simulink model "Ford_T3T6_ArchCnctnDigrm"  (R2016b)
settings: Solver=FixedStepDiscrete  StartTime=0.0  StopTime=10.0  RelTol=1e-3  EnableMultiTasking=on
libraries: canmsglib x15
(part 15 of 15)

== system Ford_T3T6_ArchCnctnDigrm/Monitor System/Measured Signals/ProcessHandwheelTorqueSignal/ES229C_HwTqCorrln ==
  HwTqA : Inport
  HwTqAQlfr : Inport  Port=2
  HwTqARollgCntr : Inport  Port=3
  HwTqB : Inport  Port=4
  HwTqBQlfr : Inport  Port=5
  HwTqBRollgCntr : Inport  Port=6
  HwTqC : Inport  Port=7
  HwTqCQlfr : Inport  Port=8
  HwTqCRollgCntr : Inport  Port=9
  HwTqD : Inport  Port=10
  HwTqDQlfr : Inport  Port=11
  HwTqDRollgCntr : Inport  Port=12
  FltInj_u08 : Inport  Port=13
  GetNtcQlfrSts : Inport  Port=14
  SetNtcSts : Inport  Port=15
  HwTqCorrlnSts : Outport
  HwTqIdptSig : Outport  Port=2

== system Ford_T3T6_ArchCnctnDigrm/Vehicle Com/Rx Messages/Acc Pedal Posn/MM062A_FordMsg204BusHiSpd ==
  AccrPedlPosnSts : Inport
  AccrPedlPosnStsQlyFac : Inport  Port=2
  CanDtcInhb : Inport  Port=3
  EngSpd : Inport  Port=4
  EpsLifeCycMod : Inport  Port=5
  TrlrBackUpAssiEnad : Inport  Port=6
  GetRefTmr100MicroSec32bit : Inport  Port=7
  GetTiSpan100MicroSec32bit : Inport  Port=8
  SetNtcSts : Inport  Port=9
  FordVehAccrPedlPosnStsQlyFac : Outport
  FordVehAccrPedlPosnStsQlyFacRaw : Outport  Port=2
  FordVehAccrPedlPosnStsRaw : Outport  Port=3
  FordVehAccrPedlPosnStsVld : Outport  Port=4
  FordVehEngSpdRaw : Outport  Port=5
  FordVehEngSpdVld : Outport  Port=6
  FordMsg204HiSpdBusClrDiagcSrv : Outport  Port=7
  FordMsg204HiSpdBusSerlComInpDi : Outport  Port=8

== system Ford_T3T6_ArchCnctnDigrm/Vehicle Com/Rx Messages/Ambient Temperature/MM078A_FordMsg41ABusHiSpd ==
  ClrDiagcFlgProxy : Inport
  FordCanDtcInhb : Inport  Port=2
  FordEpsLifeCycMod : Inport  Port=3
  Ford_Outside_Air_Temp_Stat : Inport  Port=4
  GetRefTmr100MicroSec32bit : Inport  Port=5
  GetTiSpan100MicroSec32bit : Inport  Port=6
  SetNtcSts : Inport  Port=7
  FordVehOutdAirT : Outport
  FordVehOutdAirTRaw : Outport  Port=2
  ComIPduCallout_Climate_Control_Data_FD1 : Outport  Port=3
  ComTimeoutNotification_Outside_Air_Temp_Stat : Outport  Port=4

== system Ford_T3T6_ArchCnctnDigrm/Vehicle Com/Rx Messages/Brake Data/MM052A_FordMsg07DBusHiSpd ==
  ClrDiagcFlgProxy : Inport
  FordBrkOscnRednEnad : Inport  Port=2
  FordCanDtcInhb : Inport  Port=3
  FordEpsLifeCycMod : Inport  Port=4
  FordTrlrBackUpAssiEnad : Inport  Port=5
  Ford_BrkTot_Tq_Actl : Inport  Port=6
  Ford_VehVertComp_A_Actl : Inport  Port=7
  GetRefTmr100MicroSec32bit : Inport  Port=8
  GetTiSpan100MicroSec32bit : Inport  Port=9
  SetNtcSts : Inport  Port=10
  FordVehActBrkTqRaw : Outport
  FordVehBrkTqVld : Outport  Port=2
  FordVehVertACmpdRaw : Outport  Port=3
  FordVehVertAVld : Outport  Port=4
  ComIPduCallout_BrakeSnData_4_FD1 : Outport  Port=5
  ComTimeoutNotification_BrkTot_Tq_Actl : Outport  Port=6

== system Ford_T3T6_ArchCnctnDigrm/Vehicle Com/Rx Messages/Brake Data/MM058A_FordMsg165BusHiSpd ==
  ClrDiagcFlgProxy : Inport
  FordCanDtcInhb : Inport  Port=2
  FordEpsLifeCycMod : Inport  Port=3
  FordTrlrBackupAssiEnad : Inport  Port=4
  Ford_BpedDrvAppl_D_Actl1 : Inport  Port=5
  Ford_BpedDrvAppl_D_Qf1 : Inport  Port=6
  GetRefTmr100MicroSec32bit : Inport  Port=7
  GetTiSpan100MicroSec32bit : Inport  Port=8
  SetNtcSts : Inport  Port=9
  FordVehBrkPedlAppld : Outport
  FordVehBrkPedlAppldQlyFac : Outport  Port=2
  FordVehBrkPedlVld : Outport  Port=3
  ComIPduCallout_EngBrakeData_FD1 : Outport  Port=4
  ComTimeoutNotification_BpedDrvAppl_D_Actl : Outport  Port=5

== system Ford_T3T6_ArchCnctnDigrm/Vehicle Com/Rx Messages/Brake Data/MM063A_FordMsg213BusHiSpd ==
  ClrDiagcFlgProxy : Inport
  FordBrkOscnRednEnad : Inport  Port=2
  FordCanDtcInhb : Inport  Port=3
  FordEpsLifeCycMod : Inport  Port=4
  FordEvasSteerAssiEnad : Inport  Port=5
  FordLaneCentrAssiEnad : Inport  Port=6
  FordLaneDetnWarnEnad : Inport  Port=7
  FordLkaEnad : Inport  Port=8
  FordTrfcJamAssiEnad : Inport  Port=9
  Ford_AbsActv_B_Actl1 : Inport  Port=10
  Ford_CmbbBrkDis_B_Actl1 : Inport  Port=11
  Ford_CmbbDeny_B_ActlBrk1 : Inport  Port=12
  Ford_StabCtlBrkActv_B_Actl1 : Inport  Port=13
  GetRefTmr100MicroSec32bit : Inport  Port=14
  GetTiSpan100MicroSec32bit : Inport  Port=15
  SetNtcSts : Inport  Port=16
  FordVehAbsActv : Outport
  FordVehAbsEscStsVld : Outport  Port=2
  FordVehCllsnMtgtnByBrkgDenied : Outport  Port=3
  FordVehCllsnMtgtnByBrkgDisad : Outport  Port=4
  FordVehEscActv : Outport  Port=5
  ComIPduCallout_DesiredTorqBrk_FD1 : Outport  Port=6
  ComTimeoutNotification_CmbbDeny_B_ActlBrk : Outport  Port=7

== system Ford_T3T6_ArchCnctnDigrm/Vehicle Com/Rx Messages/Brake Data/MM077A_FordMsg415BusHiSpd ==
  ClrDiagcFlgProxy : Inport
  FordAbsPrsnt : Inport  Port=2
  FordCanDtcInhb : Inport  Port=3
  FordEpsLifeCycMod : Inport  Port=4
  FordTrlrBackupAssiEnad : Inport  Port=5
  Ford_LsmcBrkDecel_D_Stat1 : Inport  Port=6
  Ford_VehVActlBrk_D_Qf1 : Inport  Port=7
  Ford_VehVActlBrk_No_Cnt : Inport  Port=8
  Ford_VehVActlBrk_No_Cs : Inport  Port=9
  Ford_Veh_V_ActlBrk : Inport  Port=10
  GetRefTmr100MicroSec32bit : Inport  Port=11
  GetTiSpan100MicroSec32bit : Inport  Port=12
  SetNtcSts : Inport  Port=13
  FordVehLoSpdMtnCtrlBrkSprtSts : Outport
  FordVehLoSpdMtnCtrlBrkSprtStsRaw : Outport  Port=2
  FordVehLoSpdMtnCtrlBrkSprtVld : Outport  Port=3
  FordVehSpdBrkModl : Outport  Port=4
  FordVehSpdBrkModlLoQlyVld : Outport  Port=5
  FordVehSpdBrkModlRaw : Outport  Port=6
  FordVehSpdBrkModlVld : Outport  Port=7
  FordVehSpdChksBrkModl : Outport  Port=8
  FordVehSpdCntrBrkModl : Outport  Port=9
  FordVehSpdQlyFacBrkModl : Outport  Port=10
  ComIPduCallout_BrakeSysFeatures_FD1 : Outport  Port=11
  ComTimeoutNotification_Veh_V_ActlBrk : Outport  Port=12

== system Ford_T3T6_ArchCnctnDigrm/Vehicle Com/Rx Messages/Evasive Steer Assist/MM075A_FordMsg3D7BusHiSpd ==
  ClrDiagcFlgProxy : Inport
  FordCanDtcInhb : Inport  Port=2
  FordEpsLifeCycMod : Inport  Port=3
  FordEvasSteerAssiEnad : Inport  Port=4
  Ford_CmbbObjClass_D_Stat1 : Inport  Port=5
  Ford_CmbbObjColl_T_Actl : Inport  Port=6
  Ford_CmbbObjConfdnc_D_Stat1 : Inport  Port=7
  Ford_CmbbObjDistLat_L_Actl : Inport  Port=8
  Ford_CmbbObjDistLong_L_Actl : Inport  Port=9
  Ford_CmbbObjRelLat_V_Actl : Inport  Port=10
  Ford_CmbbObjRelLong_V_Actl : Inport  Port=11
  Ford_EsaEnbl_D2_Rq1 : Inport  Port=12
  GetRefTmr100MicroSec32bit : Inport  Port=13
  GetTiSpan100MicroSec32bit : Inport  Port=14
  SetNtcSts : Inport  Port=15
  FordVehCllsnMtgtnByBrkgLatDstRaw : Outport
  FordVehCllsnMtgtnByBrkgLgtDstRaw : Outport  Port=2
  FordVehCllsnMtgtnByBrkgObjDataConfLvlRaw : Outport  Port=3
  FordVehCllsnMtgtnByBrkgObjTypClassnRaw : Outport  Port=4
  FordVehCllsnMtgtnByBrkgRelLatVelRaw : Outport  Port=5
  FordVehCllsnMtgtnByBrkgRelLgtVelRaw : Outport  Port=6
  FordVehCllsnMtgtnByBrkgTiToCllsnRaw : Outport  Port=7
  FordVehEvasSteerAssiEnadReqRaw : Outport  Port=8
  FordVehEvasSteerAssiImgProcrModlAVld : Outport  Port=9
  ComIPduCallout_Steer_Assist_Data_FD1 : Outport  Port=10
  ComTimeoutNotification_EsaEnbl_D2_Rq : Outport  Port=11

== system Ford_T3T6_ArchCnctnDigrm/Vehicle Com/Rx Messages/Evasive Steer Assist/MM134A_FordMsg2FDBusHiSpd ==
  ClrDiagcFlgProxy : Inport
  FordCanDtcInhb : Inport  Port=2
  FordEpsLifeCycMod : Inport  Port=3
  FordInvldMsgDiagcInhb : Inport  Port=4
  FordMfgDiagcInhb : Inport  Port=5
  FordMissMsgDiagcInhb : Inport  Port=6
  FordTrlrBackupAssiEnad : Inport  Port=7
  Ford_EsaOn_B_Rq : Inport  Port=8
  GetRefTmr100MicroSec32bit : Inport  Port=9
  GetTiSpan100MicroSec32bit : Inport  Port=10
  SetNtcSts : Inport  Port=11
  FordVehEvasSteerAssiReq : Outport
  FordVehEvasSteerAssiReqVld : Outport  Port=2
  ComIPduCallout_Mc_Send_Signals_2_FD1 : Outport  Port=3
  ComTimeoutNotification_EsaOn_B_Rq : Outport  Port=4

== system Ford_T3T6_ArchCnctnDigrm/Vehicle Com/Rx Messages/Lane Keep Asssist/MM073A_FordMsg3CABusHiSpd ==
  ClrDiagcFlgProxy : Inport
  FordCanDtcInhb : Inport  Port=2
  FordEpsLifeCycMod : Inport  Port=3
  FordLaneDetnWarnEnad : Inport  Port=4
  FordLaneKeepAssiEnad : Inport  Port=5
  Ford_LaCurvature_No_Calc : Inport  Port=6
  Ford_LaRampType_B_Req1 : Inport  Port=7
  Ford_LaRefAng_No_Req : Inport  Port=8
  Ford_LdwActvIntns_D_Req1 : Inport  Port=9
  Ford_LdwActvStats_D_Req1 : Inport  Port=10
  Ford_LkaActvStats_D2_Req1 : Inport  Port=11
  GetRefTmr100MicroSec32bit : Inport  Port=12
  GetTiSpan100MicroSec32bit : Inport  Port=13
  SetNtcSts : Inport  Port=14
  FordVehLaneAssiImgProcgModlAVld : Outport
  FordVehLaneDetnWarnInten : Outport  Port=2
  FordVehLaneDetnWarnSts : Outport  Port=3
  FordVehLaneKeepSysCrvt : Outport  Port=4
  FordVehLaneKeepSysCrvtRaw : Outport  Port=5
  FordVehLaneKeepSysRampTyp : Outport  Port=6
  FordVehLaneKeepSysReqdAg : Outport  Port=7
  FordVehLaneKeepSysReqdAgRaw : Outport  Port=8
  FordVehLaneKeepSysSts : Outport  Port=9
  ComIPduCallout_Lane_Assist_Data1_FD1 : Outport  Port=10
  ComTimeoutNotification_LaCurvature_No_Calc : Outport  Port=11

== system Ford_T3T6_ArchCnctnDigrm/Vehicle Com/Rx Messages/Lat and Long Acceleration/MM074A_FordMsg3D3BusHiSpd ==
  CanDtcInhb : Inport
  EpsLifeCycMod : Inport  Port=2
  LaneCentrAssiEnad : Inport  Port=3
  LatCtrlCrvt : Inport  Port=4
  LatCtrlCrvtRate : Inport  Port=5
  LatCtrlHandsOffDetnTqStimlsReq : Inport  Port=6
  LatCtrlPah : Inport  Port=7
  LatCtrlPahOffs : Inport  Port=8
  LatCtrlPrcsn : Inport  Port=9
  LatCtrlRampTyp : Inport  Port=10
  LatCtrlReq : Inport  Port=11
  LatCtrlRingMax : Inport  Port=12
  MissMsg3D3TiFlg : Inport  Port=13
  TrfcJamAssiEnad : Inport  Port=14
  GetRefTmr100MicroSec32bit : Inport  Port=15
  GetTiSpan100MicroSec32bit : Inport  Port=16
  SetNtcSts : Inport  Port=17
  FordVehLatCtrlCrvt : Outport
  FordVehLatCtrlCrvtRate : Outport  Port=2
  FordVehLatCtrlCrvtRateRaw : Outport  Port=3
  FordVehLatCtrlCrvtRaw : Outport  Port=4
  FordVehLatCtrlHandsOffDetnTqStimlsReq : Outport  Port=5
  FordVehLatCtrlImgProcrModlAVld : Outport  Port=6
  FordVehLatCtrlPah : Outport  Port=7
  FordVehLatCtrlPahOffs : Outport  Port=8
  FordVehLatCtrlPahOffsRaw : Outport  Port=9
  FordVehLatCtrlPahRaw : Outport  Port=10
  FordVehLatCtrlPrcsn : Outport  Port=11
  FordVehLatCtrlRampTyp : Outport  Port=12
  FordVehLatCtrlReq : Outport  Port=13
  FordVehLatCtrlRingMax : Outport  Port=14
  FordMsg3D3HiSpdBusClrDiagcSrv : Outport  Port=15
  FordMsg3D3HiSpdBusSerlComInpDi : Outport  Port=16

== system Ford_T3T6_ArchCnctnDigrm/Vehicle Com/Rx Messages/Lat and Long Acceleration/MM124A_FordMsg077BusHiSpd1 ==
  FordBrkOscnRednEnad : Inport
  FordCanDtcInhb : Inport  Port=2
  FordEpsLifeCycMod : Inport  Port=3
  FordEvasSteerAssiEnad : Inport  Port=4
  FordLaneKeepingAssiEnad : Inport  Port=5
  FordMissMsgDiagcInhb : Inport  Port=6
  FordPullDriftCmpEnad : Inport  Port=7
  FordTqSteerCmpEnad : Inport  Port=8
  FordTrlrBackupAssiEnad : Inport  Port=9
  Ford_VehLatComp_A_Actl : Inport  Port=10
  Ford_VehLongComp_A_Actl : Inport  Port=11
  Ford_VehOverGnd_V_Est : Inport  Port=12
  Ford_VehYawComp_W_Actl : Inport  Port=13
  LaneCentrAssiEnad : Inport  Port=14
  TrfcJamAssiEnad : Inport  Port=15
  GetRefTmr100MicroSec32bit : Inport  Port=16
  GetTiSpan100MicroSec32bit : Inport  Port=17
  SetNtcSts : Inport  Port=18
  FordVehLatACmpd : Outport
  FordVehLatACmpdRaw : Outport  Port=2
  FordVehLatACmpdVld : Outport  Port=3
  FordVehLgtACmpd : Outport  Port=4
  FordVehLgtACmpdRaw : Outport  Port=5
  FordVehLgtACmpdVld : Outport  Port=6
  FordVehSpdOverGnd : Outport  Port=7
  FordVehSpdOverGndRaw : Outport  Port=8
  FordVehSpdOverGndVld : Outport  Port=9
  FordVehYawRateCmpd : Outport  Port=10
  FordVehYawRateCmpdRaw : Outport  Port=11
  FordVehYawRateCmpdVld : Outport  Port=12
  ComIPduCallout_BrakeSnData_3_FD1 : Outport  Port=13
  ComTimeoutNotification_VehLatComp_A_Actl : Outport  Port=14

== system Ford_T3T6_ArchCnctnDigrm/Vehicle Com/Rx Messages/Park Assist/MM071A_FordMsg3A8BusHiSpd ==
  ClrDiagcFlgProxy : Inport
  FordApaEnad : Inport  Port=2
  FordCanDtcInhb : Inport  Port=3
  FordEpsLifeCycMod : Inport  Port=4
  FordExtAgCtrlEnad : Inport  Port=5
  FordTrlrBackUpAssiEnad : Inport  Port=6
  Ford_ApaSys_D_Stat1 : Inport  Port=7
  Ford_EPASExtAngleStatReq1 : Inport  Port=8
  Ford_ExtSteeringAngleReq2 : Inport  Port=9
  GetRefTmr100MicroSec32bit : Inport  Port=10
  GetTiSpan100MicroSec32bit : Inport  Port=11
  SetNtcSts : Inport  Port=12
  FordVehParkAidModlReqdAg : Outport
  FordVehParkAidModlReqdAgRaw : Outport  Port=2
  FordVehParkAidModlReqdAgVldInt : Outport  Port=3
  FordVehParkAidModlReqdSts : Outport  Port=4
  FordVehParkAidModlStsVld : Outport  Port=5
  FordVehParkAidModlStsVldInt : Outport  Port=6
  FordVehParkAidModlSysSt : Outport  Port=7
  ComIPduCallout_ParkAid_Data_FD1 : Outport  Port=8
  ComTimeoutNotification_EPASExtAngleStatReq : Outport  Port=9

== system Ford_T3T6_ArchCnctnDigrm/Vehicle Com/Rx Messages/Pinion Data/MM070A_FordMsg414BusHiSpd ==
  Ford_StePinOffst_An_Est : Inport
  Ford_StePinOffst_D_Stat1 : Inport  Port=2
  Ford_StePinOffst_No_Cnt : Inport  Port=3
  Ford_StePinOffst_No_Cs : Inport  Port=4
  GetRefTmr100MicroSec32bit : Inport  Port=5
  GetTiSpan100MicroSec32bit : Inport  Port=6
  FordVehSteerPinionAgOffs : Outport
  FordVehSteerPinionAgOffsRaw : Outport  Port=2
  FordVehSteerPinionAgOffsVld : Outport  Port=3
  FordVehSteerPinionOffsChks : Outport  Port=4
  FordVehSteerPinionOffsCnt : Outport  Port=5
  FordVehSteerPinionOffsSts : Outport  Port=6
  FordVehSteerPinionOffsStsRaw : Outport  Port=7
  ComIPduCallout_BrakeSnData_6_HS2 : Outport  Port=8
  ComTimeoutNotification_Ford_StePinOffst_D_Stat : Outport  Port=9

== system Ford_T3T6_ArchCnctnDigrm/Vehicle Com/Rx Messages/Steering Request Command/MM123A_FordMsg076BusHiSpd1 ==
  ClrDiagcFlgProxy : Inport
  DrvrSteerRcmdnEnad : Inport  Port=2
  FordCanDtcInhb : Inport  Port=3
  FordEpsLifeCycMod : Inport  Port=4
  Ford_DrvSte_D_Stat : Inport  Port=5
  Ford_DrvSte_Tq_Rq : Inport  Port=6
  GetRefTmr100MicroSec32bit : Inport  Port=7
  GetTiSpan100MicroSec32bit : Inport  Port=8
  SetNtcSts : Inport  Port=9
  FordVehDrvrSteerReqCmd : Outport
  FordVehDrvrSteerReqCmdVld : Outport  Port=2
  FordVehDrvrSteerReqSts : Outport  Port=3
  ComIPduCallout_BrakeSnData_5_FD1 : Outport  Port=4
  ComTimeoutNotification_DrvSte_Tq_Rq : Outport  Port=5

== system Ford_T3T6_ArchCnctnDigrm/Vehicle Com/Rx Messages/Trailer Aid/MM057A_FordMsg215BusHiSpd ==
  ClrDiagcFlgProxy : Inport
  FordCanDtcInhb : Inport  Port=2
  FordEpsLifeCycMod : Inport  Port=3
  FordTrlrBackupAssiEnad : Inport  Port=4
  Ford_TrlrAidMde_D_Rq1 : Inport  Port=5
  GetRefTmr100MicroSec32bit : Inport  Port=6
  GetTiSpan100MicroSec32bit : Inport  Port=7
  SetNtcSts : Inport  Port=8
  FordVehTrlrAidModReq : Outport
  FordVehTrlrAidModReqVld : Outport  Port=2
  ComIPduCallout_APIM_Send_Signals_2_FD1 : Outport  Port=3
  ComTimeoutNotification_TrlrAidMde_D_Rq : Outport  Port=4

== system Ford_T3T6_ArchCnctnDigrm/Vehicle Com/Rx Messages/Trailer Aid/MM069A_FordMsg3F1BusHiSpd ==
  ClrDiagcFlgProxy : Inport
  FordCanDtcInhb : Inport  Port=2
  FordEpsLifeCycMod : Inport  Port=3
  FordMfgDiagcInhb : Inport  Port=4
  FordMissMsgDiagcInhb : Inport  Port=5
  FordTrlrBackUpAssiEnad : Inport  Port=6
  Ford_TrlrAidCancl_B_Rq1 : Inport  Port=7
  GetRefTmr100MicroSec32bit : Inport  Port=8
  GetTiSpan100MicroSec32bit : Inport  Port=9
  SetNtcSts : Inport  Port=10
  FordVehTrlrAidCnclReq : Outport
  FordVehTrlrAidCnclReqVld : Outport  Port=2
  ComIPduCallout_APIM_Sen_Signals1_FD1 : Outport  Port=3
  ComTimeoutNotification_TrlrAidCancl_B_Rq : Outport  Port=4

== system Ford_T3T6_ArchCnctnDigrm/Vehicle Com/Rx Messages/Trailer Aid/MM080A_FordMsg451BusHiSpd ==
  ClrDiagcFlgProxy : Inport
  FordCanDtcInhb : Inport  Port=2
  FordEpsLifeCycMod : Inport  Port=3
  FordTrlrBackupAssiEnad : Inport  Port=4
  Ford_TrlrRvrseEnbl_D2_Stat1 : Inport  Port=5
  Ford_TrlrRvrseMsgTxt_D2_Rq : Inport  Port=6
  GetRefTmr100MicroSec32bit : Inport  Port=7
  GetTiSpan100MicroSec32bit : Inport  Port=8
  SetNtcSts : Inport  Port=9
  FordVehTrlrRvsEnaRaw : Outport
  FordVehTrlrRvsMsgTxtReqRaw : Outport  Port=2
  ImgProcgDataPrsntInt : Outport  Port=3
  ComIPduCallout_Image_Processing_Data_FD1 : Outport  Port=4
  ComTimeoutNotification_TrlrRvrseMsgTxt_D2_Rq : Outport  Port=5

== system Ford_T3T6_ArchCnctnDigrm/Vehicle Com/Rx Messages/Trailer Aid/MM083A_FordMsg457BusHiSpd ==
  ClrDiagcFlgProxy : Inport
  FordCanDtcInhb : Inport  Port=2
  FordEpsLifeCycMod : Inport  Port=3
  FordTrlrBackupAssiEnad : Inport  Port=4
  Ford_TrlrHitYaw_AnRate_Actl : Inport  Port=5
  Ford_TrlrHitchYaw_An_Actl : Inport  Port=6
  Ford_TrlrHitchYaw_D_Stat1 : Inport  Port=7
  Ford_TrlrYaw_W_Actl : Inport  Port=8
  Ford_TrlrYaw_W_Actl_D_Qf1 : Inport  Port=9
  GetRefTmr100MicroSec32bit : Inport  Port=10
  GetTiSpan100MicroSec32bit : Inport  Port=11
  SetNtcSts : Inport  Port=12
  FordVehTrlrHitchAgRateRaw : Outport
  FordVehTrlrHitchYawAgRaw : Outport  Port=2
  FordVehTrlrHitchYawSts : Outport  Port=3
  FordVehTrlrYawRateQlyFac : Outport  Port=4
  FordVehTrlrYawRateRaw : Outport  Port=5
  ComIPduCallout_TrailerAid_Stat2_FD1 : Outport  Port=6
  ComTimeoutNotification_TrlrHitchYaw_An_Actl : Outport  Port=7

== system Ford_T3T6_ArchCnctnDigrm/Vehicle Com/Rx Messages/Trailer Aid/MM086A_FordMsg443BusHiSpd ==
  ClrDiagcFlgProxy : Inport
  FordCanDtcInhb : Inport  Port=2
  FordEpsLifeCycMod : Inport  Port=3
  FordTrlrBackUpAssiEnad : Inport  Port=4
  Ford_TrlrLampCnnct_B_Actl1 : Inport  Port=5
  GetRefTmr100MicroSec32bit : Inport  Port=6
  GetTiSpan100MicroSec32bit : Inport  Port=7
  SetNtcSts : Inport  Port=8
  FordVehTrlrLampCnctnStsRaw : Outport
  ComIPduCallout_TrailerInfo_FD1 : Outport  Port=2
  ComTimeoutNotification_TrlrLampCnnct_B_Actl : Outport  Port=3

== system Ford_T3T6_ArchCnctnDigrm/Vehicle Com/Rx Messages/Trailer Aid/MM087A_FordMsg445BusHiSpd ==
  ClrDiagcFlgProxy : Inport
  FordCanDtcInhb : Inport  Port=2
  FordEpsLifeCycMod : Inport  Port=3
  FordTrlrBackUpAssiEnad : Inport  Port=4
  Ford_TrlrBrkActCnnct_B_Actl1 : Inport  Port=5
  GetRefTmr100MicroSec32bit : Inport  Port=6
  GetTiSpan100MicroSec32bit : Inport  Port=7
  SetNtcSts : Inport  Port=8
  FordVehTrlrBrkCnctnStsRaw : Outport
  ComIPduCallout_TrailerBrakeInfo_FD1 : Outport  Port=2
  ComTimeoutNotification_TrlrBrkActCnnct_B_Actl : Outport  Port=3

== system Ford_T3T6_ArchCnctnDigrm/Vehicle Com/Rx Messages/Trailer Aid/MM088A_FordMsg45ABusHiSpd ==
  ClrDiagcFlgProxy : Inport
  FordCanDtcInhb : Inport  Port=2
  FordEpsLifeCycMod : Inport  Port=3
  FordTrlrBackupAssiEnad : Inport  Port=4
  Ford_TrlrAnOffstDir_D_Mem1 : Inport  Port=5
  Ford_TrlrAxleToBmpr_L_Actl : Inport  Port=6
  Ford_TrlrIdType_D_Stat1 : Inport  Port=7
  Ford_TrlrId_No_Actl : Inport  Port=8
  Ford_TrlrRvrseCancl_B_Rq1 : Inport  Port=9
  GetRefTmr100MicroSec32bit : Inport  Port=10
  GetTiSpan100MicroSec32bit : Inport  Port=11
  SetNtcSts : Inport  Port=12
  FordVehTrlrAgOffsDirRaw : Outport
  FordVehTrlrAidIdnNrRaw : Outport  Port=2
  FordVehTrlrAxleToBmpRaw : Outport  Port=3
  FordVehTrlrBackupAssiMeasVld : Outport  Port=4
  FordVehTrlrIdnTypRaw : Outport  Port=5
  FordVehTrlrRvsCnclReqRaw : Outport  Port=6
  TrlrAidDataPrsntInt : Outport  Port=7
  ComIPduCallout_TrailerAid_Data_FD1 : Outport  Port=8
  ComTimeoutNotification_TrlrId_No_Actl : Outport  Port=9

== system Ford_T3T6_ArchCnctnDigrm/Vehicle Com/Rx Messages/Trailer Aid/MM090A_FordMsg459BusHiSpd ==
  ClrDiagcFlgProxy : Inport
  FordCanDtcInhb : Inport  Port=2
  FordEpsLifeCycMod : Inport  Port=3
  FordMfgDiagcInhb : Inport  Port=4
  FordMissMsgDiagcInhb : Inport  Port=5
  FordTrlrBackupAssiEnad : Inport  Port=6
  Ford_HitchToVehAxle_L_Calc : Inport  Port=7
  Ford_TrlrAidTrgtId_No_Actl : Inport  Port=8
  Ford_TrlrAid_An3_Actl : Inport  Port=9
  Ford_TrlrAid_AnRate2_Actl : Inport  Port=10
  Ford_TrlrAid_D2_Stat : Inport  Port=11
  Ford_TrlrRvrse_D_Stat : Inport  Port=12
  Ford_TrlrTrgtAcquire_D_Stat : Inport  Port=13
  GetRefTmr100MicroSec32bit : Inport  Port=14
  GetTiSpan100MicroSec32bit : Inport  Port=15
  SetNtcSts : Inport  Port=16
  FordVehTrlrAidAcqSts : Outport
  FordVehTrlrAidHitchAg : Outport  Port=2
  FordVehTrlrAidHitchAgRate : Outport  Port=3
  FordVehTrlrAidIdnVal : Outport  Port=4
  FordVehTrlrAidTrakgSt : Outport  Port=5
  FordVehTrlrAidTrlrRvsGuidcSts : Outport  Port=6
  FordVehTrlrBallToAxle : Outport  Port=7
  FordVehTrlrHitchAgVld : Outport  Port=8
  FordVehTrlrHitchRateVld : Outport  Port=9
  FordVehTrlrTarVld : Outport  Port=10
  FordVehTrlrTrakgStVld : Outport  Port=11
  TrlrAidStsThreePrsntInt : Outport  Port=12
  ComIPduCallout_TrailerAidStat3_FD1 : Outport  Port=13
  ComTimeoutNotification_HitchToVehAxle_L_Calc : Outport  Port=14

== system Ford_T3T6_ArchCnctnDigrm/Vehicle Com/Rx Messages/Trailer Aid/MM091A_FordMsg45CBusHiSpd ==
  ClrDiagcFlgProxy : Inport
  FordCanDtcInhb : Inport  Port=2
  FordEpsLifeCycMod : Inport  Port=3
  FordMfgDiagcInhb : Inport  Port=4
  FordMissMsgDiagcInhb : Inport  Port=5
  FordTrlrBackupAssiEnad : Inport  Port=6
  Ford_TrlrAidEnbl_D2_Rq : Inport  Port=7
  Ford_TrlrAidSetup_D2_Rq : Inport  Port=8
  GetRefTmr100MicroSec32bit : Inport  Port=9
  GetTiSpan100MicroSec32bit : Inport  Port=10
  SetNtcSts : Inport  Port=11
  FordVehTrlrAidSetUpRaw : Outport
  FordVehTrlrEnaReqRaw : Outport  Port=2
  TrlrAidDataThreePrsntInt : Outport  Port=3
  ComIPduCallout_TrailerAid_Data3_FD1 : Outport  Port=4
  ComTimeoutNotification_TrlrAidEnbl_D2_Rq : Outport  Port=5

== system Ford_T3T6_ArchCnctnDigrm/Vehicle Com/Rx Messages/Trailer Aid/MM092A_FordMsg47BusHiSpd ==
  ClrDiagcFlgProxy : Inport
  FordCanDtcInhb : Inport  Port=2
  FordEpsLifeCycMod : Inport  Port=3
  FordTrlrBackUpAssiEnad : Inport  Port=4
  Ford_TrlrAidCtl_U_RqDrv1 : Inport  Port=5
  Ford_TrlrAidSwtch_D_RqDrv : Inport  Port=6
  GetRefTmr100MicroSec32bit : Inport  Port=7
  GetTiSpan100MicroSec32bit : Inport  Port=8
  SetNtcSts : Inport  Port=9
  FordVehTrlrAidKnobBtn : Outport
  FordVehTrlrAidKnobPosn : Outport  Port=2
  ComIPduCallout_TrailerInfo_2_FD1 : Outport  Port=3
  ComTimeoutNotification_TrlrAidSwtch_D_RqDrv : Outport  Port=4

== system Ford_T3T6_ArchCnctnDigrm/Vehicle Com/Rx Messages/Transmission Data/MM060A_FordMsg176BusHiSpd ==
  ClrDiagcFlgProxy : Inport
  FordCanDtcInhb : Inport  Port=2
  FordEpsLifeCycMod : Inport  Port=3
  FordInvldMsgDiagcInhb : Inport  Port=4
  FordMfgDiagcInhb : Inport  Port=5
  FordMissMsgDiagcInhb : Inport  Port=6
  FordTrlrBackupAssiEnad : Inport  Port=7
  Ford_GearPos_D_Actl : Inport  Port=8
  Ford_TrnRng_D_Rq : Inport  Port=9
  GetRefTmr100MicroSec32bit : Inport  Port=10
  GetTiSpan100MicroSec32bit : Inport  Port=11
  SetNtcSts : Inport  Port=12
  FordVehGearPosnRaw : Outport
  FordVehGearPosnRawVldInt : Outport  Port=2
  FordVehTrsmDesGearRaw : Outport  Port=3
  FordVehTrsmDesGearRawVldInt : Outport  Port=4
  ComIPduCallout_PowertrainData_10_FD1 : Outport  Port=5
  ComTimeoutNotification_GearPos_D_Actl : Outport  Port=6

== system Ford_T3T6_ArchCnctnDigrm/Vehicle Com/Rx Messages/Transmission Data/MM061A_FordMsg202BusHiSpd ==
  ClrDiagcFlgProxy : Inport
  FordAbsPrsnt : Inport  Port=2
  FordBrkOscnRednEnad : Inport  Port=3
  FordCanDtcInhb : Inport  Port=4
  FordEpsLifeCycMod : Inport  Port=5
  FordInvldMsgDiagcInhb : Inport  Port=6
  FordMfgDiagcInhb : Inport  Port=7
  FordMissMsgDiagcInhb : Inport  Port=8
  FordTqSteerCmpEnad : Inport  Port=9
  FordTrlrBackupAssiEnad : Inport  Port=10
  Ford_GearRvrse_D_Actl1 : Inport  Port=11
  Ford_VehVActlEng_D_Qf1 : Inport  Port=12
  Ford_VehVActlEng_No_Cnt : Inport  Port=13
  Ford_VehVActlEng_No_Cs : Inport  Port=14
  Ford_VehVTrlrAid_B_Avail1 : Inport  Port=15
  Ford_Veh_V_ActlEng : Inport  Port=16
  GetRefTmr100MicroSec32bit : Inport  Port=17
  GetTiSpan100MicroSec32bit : Inport  Port=18
  SetNtcSts : Inport  Port=19
  FordVehGearRvsSts : Outport
  FordVehGearRvsStsRaw : Outport  Port=2
  FordVehGearRvsStsVld : Outport  Port=3
  FordVehSpdChksEngModl : Outport  Port=4
  FordVehSpdCntrEngModl : Outport  Port=5
  FordVehSpdEngModLoQlyVld : Outport  Port=6
  FordVehSpdEngModl : Outport  Port=7
  FordVehSpdEngModlRaw : Outport  Port=8
  FordVehSpdEngModlVld : Outport  Port=9
  FordVehSpdQlyFacEngModl : Outport  Port=10
  FordVehTrlrAidAvl : Outport  Port=11
  FordVehTrlrAidAvlRaw : Outport  Port=12
  FordVehTrlrBackupAssiAvlVld : Outport  Port=13
  ComIPduCallout_EngVehicleSpThrottle2_HS2 : Outport  Port=14
  ComTimeoutNotification_Ford_VehVActlEng_D_Qf : Outport  Port=15

== system Ford_T3T6_ArchCnctnDigrm/Vehicle Com/Rx Messages/Transmission Data/MM066A_FordMsg230BusHiSpd ==
  ClrDiagcFlgProxy : Inport
  FordCanDtcInhb : Inport  Port=2
  FordEpsLifeCycMod : Inport  Port=3
  FordTrlrBackupAssiEnad : Inport  Port=4
  Ford_GearLvrPos_D_Actl1 : Inport  Port=5
  GetRefTmr100MicroSec32bit : Inport  Port=6
  GetTiSpan100MicroSec32bit : Inport  Port=7
  SetNtcSts : Inport  Port=8
  FordVehGearLvrPosn : Outport
  FordVehGearLvrPosnVldInt : Outport  Port=2
  ComIPduCallout_TransGearData_FD1 : Outport  Port=3
  ComTimeoutNotification_GearLvrPos_D_Actl : Outport  Port=4

== system Ford_T3T6_ArchCnctnDigrm/Vehicle Com/Rx Messages/Vehicle Data/MM054A_FordMsg083BusHiSpd ==
  ClrDiagcFlgProxy : Inport
  FordCanDtcInhb : Inport  Port=2
  FordEpsLifeCycMod : Inport  Port=3
  FordLaneDetnWarnEnad : Inport  Port=4
  Ford_TurnLghtSwtch_D_Stat1 : Inport  Port=5
  GetRefTmr100MicroSec32bit : Inport  Port=6
  GetTiSpan100MicroSec32bit : Inport  Port=7
  SetNtcSts : Inport  Port=8
  FordVehTurnSigSwtStsRaw : Outport
  FordVehTurnSigVld : Outport  Port=2
  ComIPduCallout_Steering_Data_FD1 : Outport  Port=3
  ComTimeoutNotification_TurnLghtSwtch_D_Stat : Outport  Port=4

== system Ford_T3T6_ArchCnctnDigrm/Vehicle Com/Rx Messages/Vehicle Data/MM072A_FordMsg3B3BusHiSpd ==
  ClrDiagcFlgProxy : Inport
  FordCanDtcInhb : Inport  Port=2
  FordEpsLifeCycMod : Inport  Port=3
  Ford_Ignition_Status1 : Inport  Port=4
  Ford_LifeCycMde_D_Actl1 : Inport  Port=5
  GetRefTmr100MicroSec32bit : Inport  Port=6
  GetTiSpan100MicroSec32bit : Inport  Port=7
  SetNtcSts : Inport  Port=8
  FordVehIgnSts : Outport
  FordVehIgnStsVld : Outport  Port=2
  FordVehLifeCycMod : Outport  Port=3
  ComIPduCallout_BodyInfo_3_FD1 : Outport  Port=4
  ComTimeoutNotification_Ignition_Status : Outport  Port=5

== system Ford_T3T6_ArchCnctnDigrm/Vehicle Com/Rx Messages/Vehicle Data/MM076A_FordMsg40ABusHiSpd ==
  ClrDiagcFlgProxy : Inport
  FordCanDtcInhb : Inport  Port=2
  FordEpsLifeCycMod : Inport  Port=3
  Ford_VehicleGGCCData : Inport  Port=4
  GetRefTmr100MicroSec32bit : Inport  Port=5
  GetTiSpan100MicroSec32bit : Inport  Port=6
  SetNtcSts : Inport  Port=7
  FordVehGlbRealTi : Outport
  FordVehIdnNr : Outport  Port=2
  FordVehTireCircum : Outport  Port=3
  ComIPduCallout_GGCC_Config_Mgmt_ID_1_FD1 : Outport  Port=4
  ComTimeoutNotification_VehicleGGCCData : Outport  Port=5

== system Ford_T3T6_ArchCnctnDigrm/Vehicle Com/Rx Messages/Vehicle Data/MM079A_FordMsg41EBusHiSpd ==
  ClrDiagcFlgProxy : Inport
  FordCanDtcInhb : Inport  Port=2
  FordEpsLifeCycMod : Inport  Port=3
  FordSelDrvModEnad : Inport  Port=4
  Ford_SelDrvMdeChassis2_D_Rq1 : Inport  Port=5
  GetRefTmr100MicroSec32bit : Inport  Port=6
  GetTiSpan100MicroSec32bit : Inport  Port=7
  SetNtcSts : Inport  Port=8
  FordVehPenSelDrvMod : Outport
  FordVehSelDrvModChassisVld : Outport  Port=2
  ComIPduCallout_BrakeSysFeatures_3_FD1 : Outport  Port=3
  ComTimeoutNotification_SelDrvMdeChassis2_D_Rq : Outport  Port=4

== system Ford_T3T6_ArchCnctnDigrm/Vehicle Com/Rx Messages/Vehicle Data/MM081A_FordMsg430BusHiSpd ==
  ClrDiagcFlgProxy : Inport
  FordCanDtcInhb : Inport  Port=2
  FordEpsLifeCycMod : Inport  Port=3
  Ford_OdometerMasterValue : Inport  Port=4
  GetRefTmr100MicroSec32bit : Inport  Port=5
  GetTiSpan100MicroSec32bit : Inport  Port=6
  SetNtcSts : Inport  Port=7
  FordVehOdom : Outport
  ComIPduCallout_Cluster_Info1_FD1 : Outport  Port=2
  ComTimeoutNotification_OdometerMasterValue : Outport  Port=3

== system Ford_T3T6_ArchCnctnDigrm/Vehicle Com/Rx Messages/Wheel Data/MM055A_FordMsg08ABusHiSpd ==
  ClrDiagcFlgProxy : Inport
  FordActvFrntSteerPrsnt : Inport  Port=2
  FordCanDtcInhb : Inport  Port=3
  FordEpsLifeCycMod : Inport  Port=4
  Ford_SteWhlRelCalib_An_Sns : Inport  Port=5
  GetRefTmr100MicroSec32bit : Inport  Port=6
  GetTiSpan100MicroSec32bit : Inport  Port=7
  SetNtcSts : Inport  Port=8
  FordActvFrntSteerModlSteerWhlAgVldInt : Outport
  FordVehActvFrntSteerModlSteerWhlAg : Outport  Port=2
  FordVehActvFrntSteerModlSteerWhlAgRaw : Outport  Port=3
  ComIPduCallout_ActiveFrontSteering_Stat2_FD1 : Outport  Port=4
  ComTimeoutNotification_SteWhlRelCalib_An_Sns : Outport  Port=5

== system Ford_T3T6_ArchCnctnDigrm/Vehicle Com/Rx Messages/Wheel Data/MM059A_FordMsg167BusHiSpd ==
  ClrDiagcFlgProxy : Inport
  FordBrkOscnRednEnad : Inport  Port=2
  FordCanDtcInhb : Inport  Port=3
  FordEpsLifeCycMod : Inport  Port=4
  FordInvldMsgDiagcInhb : Inport  Port=5
  FordMfgDiagcInhb : Inport  Port=6
  FordMissMsgDiagcInhb : Inport  Port=7
  FordTqSteerCmpEnad : Inport  Port=8
  FordTrlrBackUpAssiEnad : Inport  Port=9
  Ford_ElPw_D_Stat1 : Inport  Port=10
  Ford_ElPw_D_StatStrtStop1 : Inport  Port=11
  Ford_PrplWhlTot2_Tq_Actl : Inport  Port=12
  Ford_PwPckTq_D_Stat1 : Inport  Port=13
  GetRefTmr100MicroSec32bit : Inport  Port=14
  GetTiSpan100MicroSec32bit : Inport  Port=15
  SetNtcSts : Inport  Port=16
  FordVehElecPwrStrtStopSts : Outport
  FordVehElecPwrSts : Outport  Port=2
  FordVehPrpnWhlTq : Outport  Port=3
  FordVehPrpnWhlTqRaw : Outport  Port=4
  FordVehPrpnWhlTqVld : Outport  Port=5
  FordVehPwrpkTqSts : Outport  Port=6
  ComIPduCallout_VehicleOperatingModes_HS2 : Outport  Port=7
  ComTimeoutNotification_PwPckTq_D_Stat : Outport  Port=8

== system Ford_T3T6_ArchCnctnDigrm/Vehicle Com/Rx Messages/Wheel Data/MM064A_FordMsg216BusHiSpd ==
  ClrDiagcFlgProxy : Inport
  FordBrkOscnRednEnad : Inport  Port=2
  FordCanDtcInhb : Inport  Port=3
  FordEpsLifeCycMod : Inport  Port=4
  FordMfgDiagcInhb : Inport  Port=5
  FordMissMsgDiagcInhb : Inport  Port=6
  FordTqSteerCmpEnad : Inport  Port=7
  FordTrlrBackUpAssiEnad : Inport  Port=8
  Ford_WhlDirFl_D_Actl1 : Inport  Port=9
  Ford_WhlDirFr_D_Actl1 : Inport  Port=10
  Ford_WhlDirRl_D_Actl1 : Inport  Port=11
  Ford_WhlDirRr_D_Actl1 : Inport  Port=12
  Ford_WhlRotatFl_No_Cnt : Inport  Port=13
  Ford_WhlRotatFr_No_Cnt : Inport  Port=14
  Ford_WhlRotatRl_No_Cnt : Inport  Port=15
  Ford_WhlRotatRr_No_Cnt : Inport  Port=16
  GetRefTmr100MicroSec32bit : Inport  Port=17
  GetTiSpan100MicroSec32bit : Inport  Port=18
  SetNtcSts : Inport  Port=19
  FordVehFrntLeWhlCntrDirVld : Outport
  FordVehFrntLeWhlDirRaw : Outport  Port=2
  FordVehFrntLeWhlRollgCntr : Outport  Port=3
  FordVehFrntRiWhlCntrDirVld : Outport  Port=4
  FordVehFrntRiWhlDirRaw : Outport  Port=5
  FordVehFrntRiWhlRollgCntr : Outport  Port=6
  FordVehReLeWhlCntrDirVld : Outport  Port=7
  FordVehReLeWhlDirRaw : Outport  Port=8
  FordVehReLeWhlRollgCntr : Outport  Port=9
  FordVehReRiWhlCntrDirVld : Outport  Port=10
  FordVehReRiWhlDirRaw : Outport  Port=11
  FordVehReRiWhlRollgCntr : Outport  Port=12
  ComIPduCallout_WheelData_FD1 : Outport  Port=13
  ComTimeoutNotification_WhlDirFl_D_Actl : Outport  Port=14

== system Ford_T3T6_ArchCnctnDigrm/Vehicle Com/Rx Messages/Wheel Data/MM065A_FordMsg217BusHiSpd ==
  ClrDiagcFlgProxy : Inport
  FordAbsPrsnt : Inport  Port=2
  FordActvNiblCtrlEnad : Inport  Port=3
  FordBrkOscnRednEnad : Inport  Port=4
  FordCanDtcInhb : Inport  Port=5
  FordEpsLifeCycMod : Inport  Port=6
  FordTqSteerCmpEnad : Inport  Port=7
  FordTrlrBackupAssiEnad : Inport  Port=8
  Ford_WhlFl_W_Meas : Inport  Port=9
  Ford_WhlFr_W_Meas : Inport  Port=10
  Ford_WhlRl_W_Meas : Inport  Port=11
  Ford_WhlRr_W_Meas : Inport  Port=12
  GetRefTmr100MicroSec32bit : Inport  Port=13
  GetTiSpan100MicroSec32bit : Inport  Port=14
  SetNtcSts : Inport  Port=15
  FordVehFrntLeWhlSpd : Outport
  FordVehFrntLeWhlSpdRaw : Outport  Port=2
  FordVehFrntLeWhlSpdVld : Outport  Port=3
  FordVehFrntRiWhlSpd : Outport  Port=4
  FordVehFrntRiWhlSpdRaw : Outport  Port=5
  FordVehFrntRiWhlSpdVld : Outport  Port=6
  FordVehReLeWhlSpd : Outport  Port=7
  FordVehReLeWhlSpdRaw : Outport  Port=8
  FordVehReLeWhlSpdVld : Outport  Port=9
  FordVehReRiWhlSpd : Outport  Port=10
  FordVehReRiWhlSpdRaw : Outport  Port=11
  FordVehReRiWhlSpdVld : Outport  Port=12
  ComIPduCallout_WheelSpeed_FD1 : Outport  Port=13
  ComTimeoutNotification_WhlFl_W_Meas : Outport  Port=14

== system Ford_T3T6_ArchCnctnDigrm/Vehicle Com/Rx Messages/Yaw Rate/MM056A_FordMsg091BusHiSpd ==
  ClrDiagcFlgProxy : Inport
  FordCanDtcInhb : Inport  Port=2
  FordEpsLifeCycMod : Inport  Port=3
  FordInvldMsgDiagcInhb : Inport  Port=4
  FordMfgDiagcInhb : Inport  Port=5
  FordMissMsgDiagcInhb : Inport  Port=6
  FordTrlrBackupAssiEnad : Inport  Port=7
  Ford_VehYaw_W_Actl : Inport  Port=8
  FordLaneCentrAssiEnad : Inport  Port=9
  FordTrfcJamAssiEnad : Inport  Port=10
  GetRefTmr100MicroSec32bit : Inport  Port=11
  GetTiSpan100MicroSec32bit : Inport  Port=12
  SetNtcSts : Inport  Port=13
  FordVehYawRate : Outport
  FordVehYawRateRaw : Outport  Port=2
  FordVehYawRateRawVld : Outport  Port=3
  ComIPduCallout_Yaw_Data_FD1 : Outport  Port=4
  ComTimeoutNotification_VehYaw_W_Actl : Outport  Port=5

== system Ford_T3T6_ArchCnctnDigrm/Vehicle Com/Rx Messages/Yaw Rate/MM082A_FordMsg452BusHiSpd ==
  ClrDiagcFlgProxy : Inport  OutMin=[0]  OutMax=[1]  OutDataTypeStr=uint8  Unit=Cnt
  FordCanDtcInhb : Inport  Port=2  OutMin=[0]  OutMax=[1]  OutDataTypeStr=boolean  Unit=Cnt
  FordEpsLifeCycMod : Inport  Port=3  OutMin=[0]  OutMax=[1]  OutDataTypeStr=boolean  Unit=Cnt
  FordInvldMsgDiagcInhb : Inport  Port=4  OutMin=[0]  OutMax=[1]  OutDataTypeStr=boolean  Unit=Cnt
  FordMfgDiagcInhb : Inport  Port=5  OutMin=[0]  OutMax=[1]  OutDataTypeStr=boolean  Unit=Cnt
  FordMissMsgDiagcInhb : Inport  Port=6  OutMin=[0]  OutMax=[1]  OutDataTypeStr=boolean  Unit=Cnt
  FordTrlrBackupAssiEnad : Inport  Port=7  OutMin=[0]  OutMax=[1]  OutDataTypeStr=boolean  Unit=Cnt
  Ford_TrlrSnsId_No_Act : Inport  Port=8  OutMin=[0]  OutMax=[255]  OutDataTypeStr=uint8  Unit=Cnt
  GetRefTmr100MicroSec32bit : Inport  Port=9  OutMin=[[]]  OutMax=[[]]
  GetTiSpan100MicroSec32bit : Inport  Port=10  OutMin=[[]]  OutMax=[[]]
  SetNtcSts : Inport  Port=11  OutMin=[[]]  OutMax=[[]]
  FordVehYawRateSnsrIdyHi : Outport  OutMin=[0]  OutMax=[4294967295]  OutDataTypeStr=uint32  Unit=Cnt
  FordVehYawRateSnsrIdyLo : Outport  Port=2  OutMin=[0]  OutMax=[4294967295]  OutDataTypeStr=uint32  Unit=Cnt
  ComIPduCallout_TrailerAid_Stat1_FD1 : Outport  Port=3  OutMin=[[]]  OutMax=[[]]
  ComTimeoutNotification_TrlrSnsId_No_Actl : Outport  Port=4  OutMin=[[]]  OutMax=[[]]

== system Ford_T3T6_ArchCnctnDigrm/Vehicle Com/Rx Messages/Yaw Rate/MM089A_FordMsg4B0BusHiSpd ==
  ClrDiagcFlgProxy : Inport
  FordBrkOscnRednEnad : Inport  Port=2
  FordCanDtcInhb : Inport  Port=3
  FordEpsLifeCycMod : Inport  Port=4
  FordEvasSteerAssiEnad : Inport  Port=5
  FordInvldMsgDiagcInhb : Inport  Port=6
  FordLaneCentrAssiEnad : Inport  Port=7
  FordMfgDiagcInhb : Inport  Port=8
  FordMissMsgDiagcInhb : Inport  Port=9
  FordTqSteerCmpEnad : Inport  Port=10
  Ford_YawStabilityIndex : Inport  Port=11
  LaneDetnWarnEnad : Inport  Port=12
  LaneKeepAssiEnad : Inport  Port=13
  TrfcJamAssiEnad : Inport  Port=14
  GetRefTmr100MicroSec32bit : Inport  Port=15
  GetTiSpan100MicroSec32bit : Inport  Port=16
  SetNtcSts : Inport  Port=17
  FordVehYawStabyRaw : Outport
  FordVehYawStabyVld : Outport  Port=2
  ComIPduCallout_ABS_BrkBst_Data_FD1 : Outport  Port=3
  ComTimeoutNotification_YawStabilityIndex : Outport  Port=4

== system Ford_T3T6_ArchCnctnDigrm/Generate Steering Command/Openloop Steering Command/GenerateSteeringCommand/Assist/SF001A_Assi ==
  AssiCmdBasSca : Inport
  AssiLnrGain : Inport  Port=2
  AssiLnrGainEna : Inport  Port=3
  HwTq : Inport  Port=4
  HwTqHysOvrl : Inport  Port=5
  HwTqOvrl : Inport  Port=6
  ThermLimSlowFilMax : Inport  Port=7
  VehSpd : Inport  Port=8
  WhlImbRejctnAmp : Inport  Port=9
  FltInj_f32 : Inport  Port=10
  AssiCmdBas : Outport

== system Ford_T3T6_ArchCnctnDigrm/Generate Steering Command/Openloop Steering Command/GenerateSteeringCommand/Assist/SF012A_HysCmp ==
  AssiCmdBas : Inport
  AssiMechT : Inport  Port=2
  HwTq : Inport  Port=3
  HysCmpCmdDi : Inport  Port=4
  SysFricOffs : Inport  Port=5
  VehSpd : Inport  Port=6
  WhlImbRejctnAmp : Inport  Port=7
  HwTqOvrl : Inport  Port=8
  FltInj_f32 : Inport  Port=9
  HysCmpCmd : Outport

== system Ford_T3T6_ArchCnctnDigrm/Generate Steering Command/Openloop Steering Command/GenerateSteeringCommand/Assist/SF028A_AssiHiFrq ==
  HwTq : Inport
  VehSpd : Inport  Port=2
  WhlImbRejctnAmp : Inport  Port=3
  AssiHiFrqCmd : Outport

== system Ford_T3T6_ArchCnctnDigrm/Generate Steering Command/Openloop Steering Command/GenerateSteeringCommand/Assist/SF029A_StabyCmp ==
  AssiCmdBasSca : Inport
  AssiCmdSum : Inport  Port=2
  AssiPahLimrActv : Inport  Port=3
  HwTq : Inport  Port=4
  VehSpd : Inport  Port=5
  FltInj_f32 : Inport  Port=6
  AssiCmd : Outport

== system Ford_T3T6_ArchCnctnDigrm/Generate Steering Command/Openloop Steering Command/GenerateSteeringCommand/Assist/SF034B_AssiPahSum ==
  AssiCmdBas : Inport
  AssiHiFrqCmd : Inport  Port=2
  HysCmpCmd : Inport  Port=3
  AssiCmdSum : Outport

== system Ford_T3T6_ArchCnctnDigrm/Generate Steering Command/Openloop Steering Command/GenerateSteeringCommand/Damping/SF003A_Dampg ==
  AssiCmdBas : Inport
  AssiMechT : Inport  Port=2
  DampgCmdBasDi : Inport  Port=3
  DampgCmdOvrl : Inport  Port=4
  DampgCmdSca : Inport  Port=5
  HwTq : Inport  Port=6
  MotVelCrf : Inport  Port=7
  VehSpd : Inport  Port=8
  FltInj_f32 : Inport  Port=9
  DampgCmdBas : Outport

== system Ford_T3T6_ArchCnctnDigrm/Generate Steering Command/Openloop Steering Command/GenerateSteeringCommand/Damping/SF014A_InertiaCmpVel ==
  AssiCmdBas : Inport
  HwTq : Inport  Port=2
  InertiaCmpDecelGainDi : Inport  Port=3
  InertiaCmpVelCmdDi : Inport  Port=4
  MotVelCrf : Inport  Port=5
  VehLgtA : Inport  Port=6
  VehSpd : Inport  Port=7
  WhlImbRejctnAmp : Inport  Port=8
  FltInj_f32 : Inport  Port=9
  InertiaCmpVelCmd : Outport

== system Ford_T3T6_ArchCnctnDigrm/Generate Steering Command/Openloop Steering Command/GenerateSteeringCommand/Damping/SF035B_DampgPahSum ==
  DampgCmdBas : Inport
  InertiaCmpVelCmd : Inport  Port=2
  DampgCmd : Outport

== system Ford_T3T6_ArchCnctnDigrm/Generate Steering Command/Openloop Steering Command/GenerateSteeringCommand/Return/SF002A_Rtn ==
  AssiMechT : Inport
  HwAg : Inport  Port=2
  HwAgAuthySca : Inport  Port=3
  HwAgRtnOffs : Inport  Port=4
  HwTq : Inport  Port=5
  HwVel : Inport  Port=6
  RtnCmdDi : Inport  Port=7
  RtnCmdDiagcDi : Inport  Port=8
  RtnCmdSca : Inport  Port=9
  RtnCmdScaServo : Inport  Port=10
  VehSpd : Inport  Port=11
  VehSpdVld : Inport  Port=12
  FltInj_f32 : Inport  Port=13
  RtnCmd : Outport

== system Ford_T3T6_ArchCnctnDigrm/Generate Steering Command/Openloop Steering Command/GenerateSteeringCommand/Return/SF036A_RtnPahFwl ==
  HwAg : Inport
  MfgEnaSt : Inport  Port=2
  RtnCmd : Inport  Port=3
  RtnCmdDi : Inport  Port=4
  VehSpd : Inport  Port=5
  SetNtcSts : Inport  Port=6
  RtnCmdLimd : Outport

== system Ford_T3T6_ArchCnctnDigrm/Generate Steering Command/Openloop Steering Command/System Protection/EoTProtection/SF016A_VehSpdLimr ==
  HwAg : Inport
  HwAgAuthy : Inport  Port=2
  HwAgEotCcw : Inport  Port=3
  HwAgEotCw : Inport  Port=4
  VehSpd : Inport  Port=5
  VehSpdMotTqLim : Outport

== system Ford_T3T6_ArchCnctnDigrm/Generate Steering Command/Openloop Steering Command/System Protection/EoTProtection/SF018A_EotProtn ==
  EotProtnDi : Inport
  HwAg : Inport  Port=2
  HwAgAuthy : Inport  Port=3
  HwAgCcwDetd : Inport  Port=4
  HwAgCwDetd : Inport  Port=5
  HwAgEotCcw : Inport  Port=6
  HwAgEotCw : Inport  Port=7
  HwTq : Inport  Port=8
  MotVelCrf : Inport  Port=9
  SysMotTqCmdSca : Inport  Port=10
  VehSpd : Inport  Port=11
  EotActvCmd : Outport
  EotAssiSca : Outport  Port=2
  EotDampgCmd : Outport  Port=3
  EotMotTqLim : Outport  Port=4

== system Ford_T3T6_ArchCnctnDigrm/Generate Steering Command/Openloop Steering Command/System Protection/EoTProtection/SF027A_EotProtnFwl ==
  EotActvCmd : Inport
  EotDampgCmd : Inport  Port=2
  EotProtnDi : Inport  Port=3
  HwAg : Inport  Port=4
  MfgEnaSt : Inport  Port=5
  MotVelCrf : Inport  Port=6
  PinionAgConf : Inport  Port=7
  VehSpd : Inport  Port=8
  SetNtcSts : Inport  Port=9
  EotActvCmdLimd : Outport
  EotDampgCmdLimd : Outport  Port=2

== system Ford_T3T6_ArchCnctnDigrm/Generate Steering Command/Openloop Steering Command/System Protection/Motor Protection/SF009A_DutyCycThermProtn ==
  DiagcStsLimdTPrfmnc : Inport
  DualEcuFltMtgtnEna : Inport  Port=2
  DutyCycThermProtnDi : Inport  Port=3
  EcuTFild : Inport  Port=4
  IgnTiOff : Inport  Port=5
  MotAndThermProtnLoaMod : Inport  Port=6
  MotCurrPeakEstimd : Inport  Port=7
  MotCurrPeakEstimdFild : Inport  Port=8
  MotFetT : Inport  Port=9
  MotMagT : Inport  Port=10
  MotVelCrf : Inport  Port=11
  MotWidgT : Inport  Port=12
  VehTiVld : Inport  Port=13
  FilStVal_GetErrorStatus : Inport  Port=14
  FilStVal_SetRamBlockStatus : Inport  Port=15
  SetNtcSts : Inport  Port=16
  DutyCycThermProtnMaxOutp : Outport
  ThermDutyCycProtnLoadDptLim : Outport  Port=2
  ThermDutyCycProtnTDptLim : Outport  Port=3
  ThermLimSlowFilMax : Outport  Port=4
  ThermMotTqLim : Outport  Port=5
  ThermRednFac : Outport  Port=6

== system Ford_T3T6_ArchCnctnDigrm/Generate Steering Command/Openloop Steering Command/System Protection/Motor Protection/SF017A_HiLoadStallLimr ==
  DualEcuFltMtgtnEna : Inport
  MotAndThermProtnLoaMod : Inport  Port=2
  MotTqCmdLimdPreStall : Inport  Port=3
  MotVelCrf : Inport  Port=4
  StallMotTqLimDi : Inport  Port=5
  StallMotTqLim : Outport
